simulink model "tv_system_lut"  (R2021b)
settings: Solver=VariableStepAuto  StartTime=0.0  StopTime=0  RelTol=1e-3
values from neighbouring files (symbols this model uses):
  gamma1 = 0.005    [main_pixloss.m]
  gamma2 = 1/(1.05*tau2)*(1/gamma1-beta/2)    [main_pixloss.m]
  lambda = 0.012    [main_pixloss.m]
  maxIter = 500    [main_pixloss.m]
  Np = 50    [main_pixloss.m]
undefined symbols (not defined in the file or in its folder): cols, gray, rows
libraries: visionsources x3, visionstatistics x2
(part 5 of 5)

== matlab function tv_system_lut/For Iterator Subsystem2/For Iterator Subsystem/Subsystem/MATLAB Function3 ==
  data: x input; out output; y input; div input
function out = l2_lut_noproduct(x,y,div)
x = min(max(x,-1),1);
y = min(max(y,-1),1);
divide_val = linspace(-1, 1, div);
[tmp1,tmp2] = meshgrid(divide_val);

truthtable = sqrt(tmp1.^2 + tmp2.^2);
truthtable = triu(truthtable);
vector_truthtable = truthtable(logical(truthtable));

% tmp1 = zeros(size(x));
% tmp2 = zeros(size(y));
truthtable_out_x = ones(size(x));
truthtable_out_y = ones(size(x));
for i = 1:numel(x)
    if x(i) < y(i)
        in_x = x(i);
        in_y = y(i);
    else
        in_x = y(i);
        in_y = x(i);
    end
    for k = 1:length(divide_val)
        if in_x > divide_val(k)
            truthtable_out_x(i) = k;
        end
        if in_y > divide_val(k)
            truthtable_out_y(i) = k;
        end
    end
end

out = cast(zeros(size(x)),'like',x);
for i = 1:numel(x)
    %out(i) = truthtable(div * truthtable_out_y(i)+truthtable_out_x(i));
    %out(i) = truthtable(truthtable_out_x(i),truthtable_out_y(i));

    n = truthtable_out_y(i);
    d = -1;
    a = div-1;
    zerosum = (1/2)*(n)*(2*a + (n-1)*(d));
    out(i) = vector_truthtable(div*truthtable_out_y(i) - zerosum + truthtable_out_x(i));
end
end

== matlab function tv_system_lut/Subsystem1/For Iterator Subsystem1/MATLAB Function ==
  data: error input; u input; erro output
function erro = fcn(error,u)

erro = norm(error(:),2) / norm(u(:),2);
